simulink model "two_jian3xie2zhen4zi3"  (Simulink 5.0)
settings: Solver=ode45  StartTime=0.0  StopTime=50.0  MaxStep=0.003  RelTol=1e-3
settings Model: LastModifiedBy=Administrator  OptimizeBlockIOStorage=off

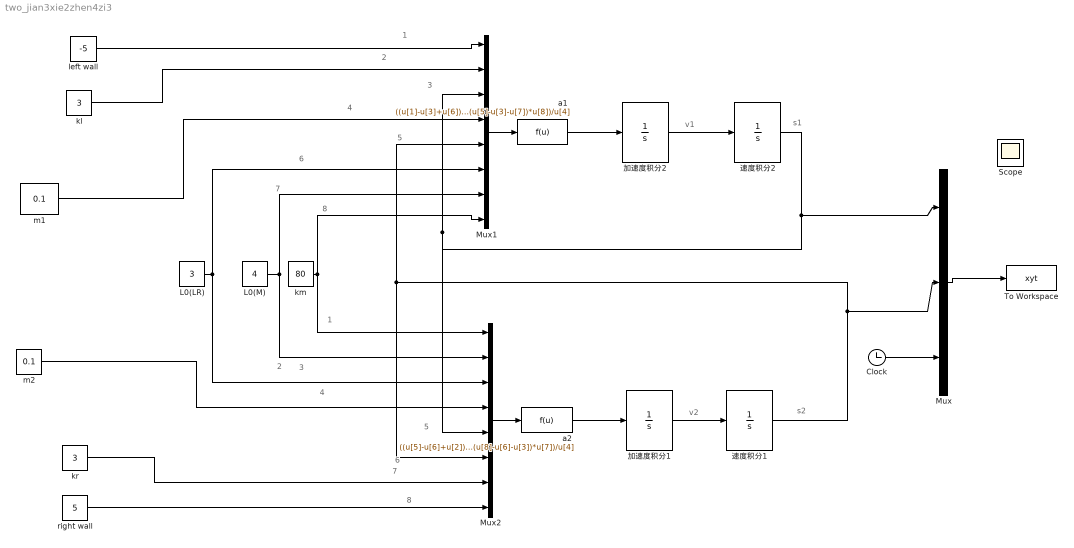
== system two_jian3xie2zhen4zi3 ==
  note: v2
  note: s2
  note: v1
  note: s1
  note: 1
  note: 2
  note: 3
  note: 4
  note: 5
  note: 6
  note: 7
  note: 8
  note: 1
  note: 2
  note: 3
  note: 4
  note: 5
  note: 6
  note: 7
  note: 8
  Clock : Clock
      settings: Decimation=10
  L0(LR) : Constant  Value=3
  "L0(M) " : Constant  Value=4
  Mux : Mux  Inputs=3
  Mux1 : Mux  Inputs=8
  Mux2 : Mux  Inputs=8
  Scope : Scope
  To Workspace : ToWorkspace  VariableName=xyt  SampleTime=-1  SaveFormat=Array
  a1 : Fcn  Expr=((u[1]-u[3]+u[6])*u[2]+(u[5]-u[3]-u[7])*u[8])/u[4]
  "a2 " : Fcn  Expr=((u[5]-u[6]+u[2])*u[1]+(u[8]-u[6]-u[3])*u[7])/u[4]
  kl : Constant  Value=3
  km : Constant  Value=80
  "kr " : Constant  Value=3
  left wall : Constant  Value=-5
  m1 : Constant  Value=0.1
  m2 : Constant  Value=0.1
  "right wall " : Constant  Value=5
  加速度积分1 : Integrator
  加速度积分2 : Integrator
  速度积分1 : Integrator
  速度积分2 : Integrator  InitialCondition=-3  ZeroCross=off
  wires:
  加速度积分1/1 -> 速度积分1/1
  加速度积分2/1 -> 速度积分2/1
  Mux1/1 -> a1/1
  a1/1 -> 加速度积分2/1
  left wall/1 -> Mux1/1
  kl/1 -> Mux1/2
  m1/1 -> Mux1/4
  L0(LR)/1 -> Mux1/6, Mux2/3
  "L0(M) "/1 -> Mux1/7, Mux2/2
  km/1 -> Mux1/8, Mux2/1
  Mux2/1 -> "a2 "/1
  "right wall "/1 -> Mux2/8
  "kr "/1 -> Mux2/7
  m2/1 -> Mux2/4
  "a2 "/1 -> 加速度积分1/1
  速度积分1/1 -> Mux1/5, Mux2/6, Mux/2
  速度积分2/1 -> Mux2/5, Mux1/3, Mux/1
  Mux/1 -> To Workspace/1
  Clock/1 -> Mux/3
